simulink model "Cascade_Fil_Realization"  (R2019b)
settings: Solver=FixedStepAuto  StartTime=0.0  StopTime=10.0  FixedStep=0.2  RelTol=1e-3
settings Model: Creator=ip  LastModifiedBy=ip
settings DataIOCC: SaveOutput=off  SaveTime=off

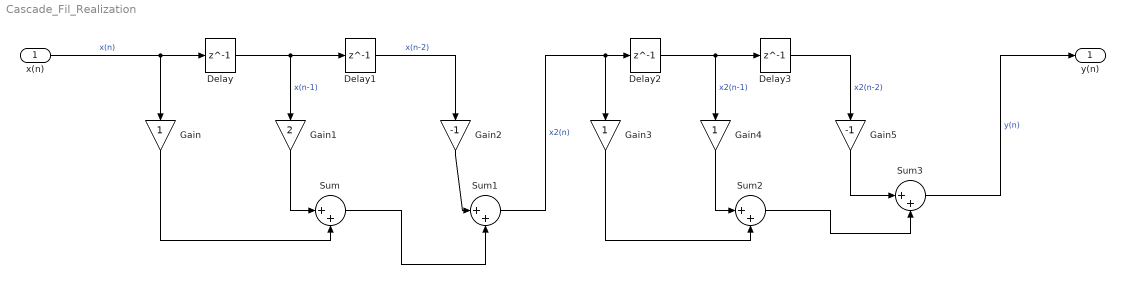
== system Cascade_Fil_Realization ==
  x(n) : Inport  OutDataTypeStr=double  PortDimensions=1  SampleTime=[0.20000000000000001,0]
  Delay{,1..3} (4 alike) : Delay  DelayLength=1
  Gain : Gain
  Gain1 : Gain  Gain=2
  Gain2 : Gain  Gain=-1
  Gain3 : Gain
  Gain4 : Gain
  Gain5 : Gain  Gain=-1
  Sum{,1..3} (4 alike) : Sum  Inputs=|++
  y(n) : Outport  OutDataTypeStr=double  PortDimensions=1  SampleTime=[0.20000000000000001,0]
  wires:
  Gain2/1 -> Sum1/1
  Sum1/1 -> Delay2/1, Gain3/1  "x2(n)"
  Sum2/1 -> Sum3/2
  Delay2/1 -> Delay3/1, Gain4/1  "x2(n-1)"
  x(n)/1 -> Delay/1, Gain/1  "x(n)"
  Gain4/1 -> Sum2/1
  Gain3/1 -> Sum2/2
  Sum/1 -> Sum1/2
  Delay/1 -> Delay1/1, Gain1/1  "x(n-1)"
  Gain5/1 -> Sum3/1
  Delay1/1 -> Gain2/1  "x(n-2)"
  Gain/1 -> Sum/2
  Delay3/1 -> Gain5/1  "x2(n-2)"
  Gain1/1 -> Sum/1
  Sum3/1 -> y(n)/1  "y(n)"
